simulink subsystem "CasADi_freetf_freefinal_6DOF"  (R2024b)
settings: Solver=VariableStepAuto  StartTime=0.0  StopTime=10.0  RelTol=1e-3
settings Model: Creator=thatf  LastModifiedBy=ishkr

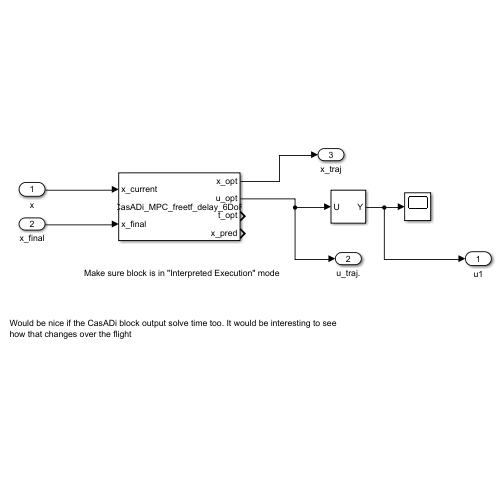
[thumbnail: Simulink's stored preview of the top-level diagram]
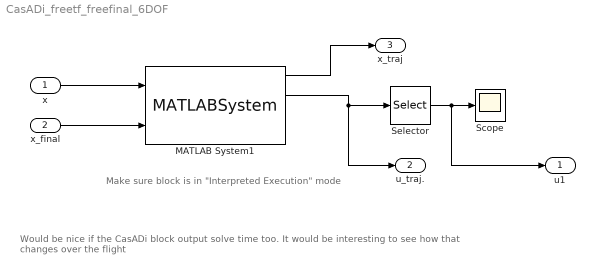
== system CasADi_freetf_freefinal_6DOF ==
  note: Make sure block is in "Interpreted Execution" mode
  note: Would be nice if the CasADi block output solve time too. It would be interesting to see how that changes over the flight
  x : Inport
  x_final : Inport  Port=2
  MATLAB System1 : MATLABSystem  System=CasADi_MPC_freetf_delay_6DoF  vehicle="Vehicle( 100000, 30, 60, deg2rad( 20 ), 800000, 2000000, Name=\"Default\" )"  max_t_step=0.5  steps=50  max_iter=400  x_initial=zeros([12 1])  x_final=[0;0;0;0;0;0;1.5707963267948966;0;0;0;0;0]  delay_time=0.1  SimulateUsing=Code generation
      mask Type: CasADi_MPC_freetf_delay_6DoF
      mask Display:
      | disp('CasADi_MPC_freetf_delay_6DoF');
      | port_label('input',1,'x_current');
      | port_label('input',2,'x_final');
      | port_label('output',1,'x_opt');
      | port_label('output',2,'u_opt');
      | port_label('output',3,'t_opt');
      | port_label('output',4,'x_pred');
  Scope : Scope
  Selector : Selector  NumberOfDimensions=2  InputPortWidth=3  IndexOptions=Index vector (dialog),Select all  Indices=[1],1  OutputSizes=1,1
  u1 : Outport
  u_traj. : Outport  Port=2
  x_traj : Outport  Port=3
  wires:
  Selector/1 -> Scope/1, u1/1
  x/1 -> MATLAB System1/1
  MATLAB System1/1 -> x_traj/1
  MATLAB System1/2 -> u_traj./1, Selector/1
  x_final/1 -> MATLAB System1/2
